simulink model "Blimp_Simulation"  (R2021a)
settings: Solver=VariableStepAuto  StartTime=0.0  StopTime=30  RelTol=1e-3
libraries: simulink x2, sim3dcameralib x1, sim3dlib x1, uavsim3dlib x1
settings Model: Creator=ritav  LastModifiedBy=ritav

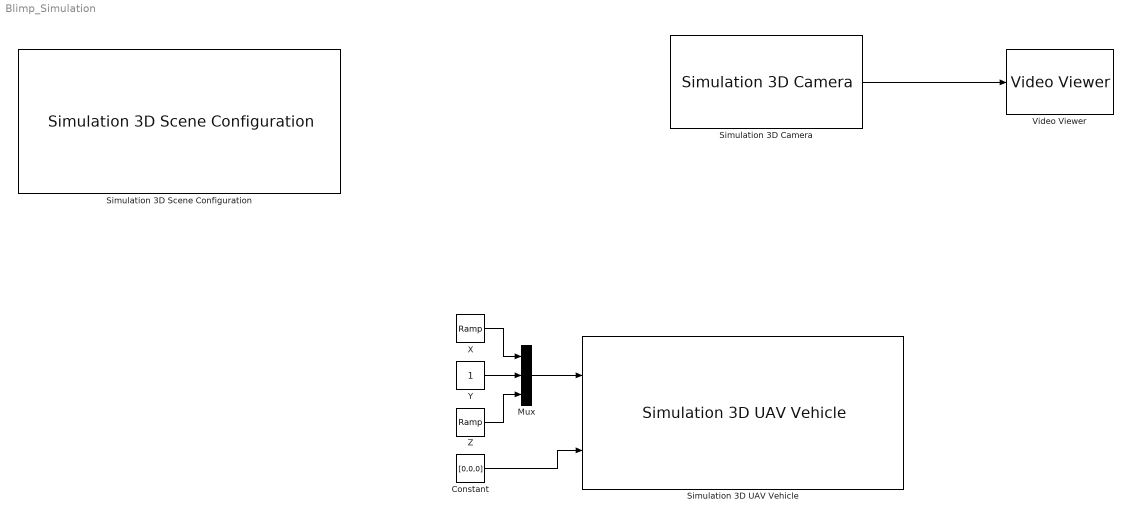
== system Blimp_Simulation ==
  Constant : Constant  Value=[0,0,0]
  Mux : Mux  Inputs=3
  Simulation 3D Camera : sim3dcameralib/Simulation 3D Camera  Priority=1  sensorTag=Sim3dSensor1  sensorId=1  sensorName=Sim3dSensor1  vehTagList={'Quadrotor1';'Scene Origin'}  vehTag=Quadrotor1  mountLoc=Origin  offsetFlag=on  tmountOffset=[0.1, 0, 0]  rmountOffset=[0, 70, 0]  FocalLength=[1109, 1109]  OpticalCenter=[640, 360]  ImageSize=[720, 1280]  RadialDistortion=[0, 0]  TangentialDistortion=[0, 0]  SensorSkew=0  DepthOutportEnabled=off  SemanticOutportEnabled=off  TransformOutportEnabled=off  SampleTime=-1  mountPoint=[0.1 0 0]  mountOrientation=[0 -70 0]  aMode=4  ID=1
      settings: SourceProductBaseCode=DR,UV,VE
  Simulation 3D Scene Configuration : sim3dlib/Simulation 3D Scene Configuration  Priority=0  ProjectFormat=Default Scenes  SceneDesc=US city block  ProjectName=C:\Program Files\Polyspace\R2021a\toolbox\shared\sim3d_projects\automotive_project\UE4\WindowsNoEditor\VehicleSimulation.exe  ScenePath=/Game/Maps/USCityBlock  vehTagList={'Quadrotor1';'Scene Origin'}  vehTag=Quadrotor1  OpVisEn=off  Ts=1/60  EnableWindow=on  EnableWeather=off  SunAltitude=40.0  SunAzimuth=90  clouds=10  wind=1  fog=0  rain=0  sensorTag=MainCamera1  sensorId=1  sensorName=MainCamera1  mountLoc=Origin  offsetFlag=off  tmountOffset=[0, 0, 0]  rmountOffset=[0, 0, 0]  HorizontalResolution=1280  VerticalResolution=720  HorizontalFOV=60  mountPoint=[0 0 0]  mountOrientation=[0 0 0]  aMode=4  ID=1
      settings: SourceProductBaseCode=DR,UV,VE
  Simulation 3D UAV Vehicle : uavsim3dlib/Simulation 3D UAV Vehicle  Priority=-1  Mesh=Quadrotor  Color=Black  ActorName=Quadrotor1  InitialTranslation=[0 0 0]  InitialRotation=[0 0 0]  SampleTime=-1  ActorType=SimulinkVehicle  ID=C  aMode=4  ActorTag=Quadrotor1
      settings: SourceProductBaseCode=UV
  Video Viewer : VideoViewer  FigPos=[1 1078 613 286]
  X : simulink/Sources/Ramp  slope=4  start=0  InitialOutput=0
  Y : Constant
  Z : simulink/Sources/Ramp  slope=3  start=0  InitialOutput=0
  wires:
  Simulation 3D Camera/1 -> Video Viewer/1
  Constant/1 -> Simulation 3D UAV Vehicle/2
  Mux/1 -> Simulation 3D UAV Vehicle/1
  Y/1 -> Mux/2
  X/1 -> Mux/1
  Z/1 -> Mux/3
